simulink model "simulacionPOLGEN"  (R2017b)
settings: Solver=VariableStepDiscrete  StartTime=0.0  StopTime=20  MaxStep=0.1  RelTol=1e-3
undefined symbols (not defined in the file): sigbuilder_block
settings Model: Creator=Ian  LastModifiedBy=Ian

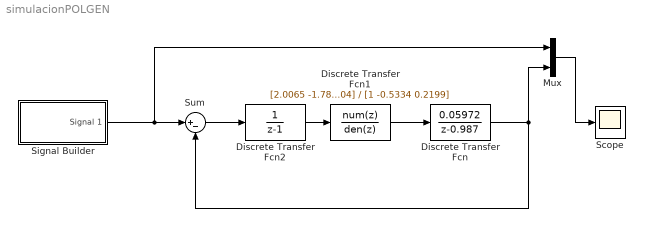
== system simulacionPOLGEN ==
  Discrete Transfer Fcn : DiscreteTransferFcn  Numerator=[0.05972]  Denominator=[1 -0.987]  SampleTime=0.1
  Discrete Transfer Fcn1 : DiscreteTransferFcn  Numerator=[2.0065 -1.7804]  Denominator=[1 -0.5334 0.2199]  SampleTime=0.1
  Discrete Transfer Fcn2 : DiscreteTransferFcn  Denominator=[1 -1]  SampleTime=0.1
  Mux : Mux  Inputs=2
  Scope : Scope
  Signal Builder : Subsystem  Tag=STV Subsys  LoadFcn=sigbuilder_block('load');  StartFcn=sigbuilder_block('start');  StopFcn=sigbuilder_block('stop');  ClipboardFcn=sigbuilder_block('clipboard');  mask(Sigbuilder block){tuvar=[0:10]}
      mask help: Simulink:masks:SigbuilderBlock_MD
      mask init:
      | if ~strcmp(get_param(bdroot(gcbh),'SimulationStatus'),'stopped') tuvar = sigbuilder_block('maskInit'); end
      settings: CopyFcn=sigbuilder_block('copy');  DeleteFcn=sigbuilder_block('delete');  ModelCloseFcn=sigbuilder_block('modelClose');  PreSaveFcn=sigbuilder_block('preSave');  PauseFcn=sigbuilder_block('pause');  ContinueFcn=sigbuilder_block('continue');  NameChangeFcn=sigbuilder_block('namechange');  OpenFcn=sigbuilder_block('open',[437.25 153 550.5 359.25 ]);  CloseFcn=sigbuilder_block('close');
      mask Display: plot(0, 0, 100, 100,[2, 2, 32, 32, 2], [68, 8, 8, 68, 68],[32, 2], [38, 38], [32, 19, 2],[53, 60, 44], [32, 17, 17, 2],[16, 16, 31, 31]);txt = getActiveGroup(gcbh);text(2, 100, txt,'verticalAlignment', 'top');
  Sum : Sum  Inputs=|+-
  wires:
  Discrete Transfer Fcn1/1 -> Discrete Transfer Fcn/1
  Discrete Transfer Fcn/1 -> Mux/2, Sum/2
  Signal Builder/1(Signal 1) -> Mux/1, Sum/1
  Mux/1 -> Scope/1
  Discrete Transfer Fcn2/1 -> Discrete Transfer Fcn1/1
  Sum/1 -> Discrete Transfer Fcn2/1

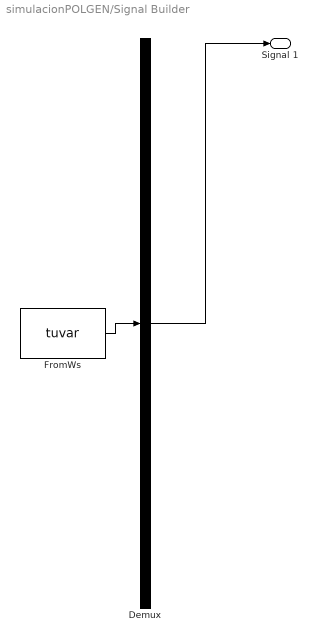
== system simulacionPOLGEN/Signal Builder ==
  Demux : Demux  Tag=STV Demux  Outputs=1
  FromWs : FromWorkspace  Tag=STV FromWs  VariableName=tuvar  SampleTime=0
      SigBuilderData=|
      | common.afterFinalStr = 'Extrapolate'
      | common.sampleTime = 0
      | dataSet.timeRange = [0 10]
      | dataSet.name = 'Group 1'
      | sbobj.Groups.Name = 'Group 1'
      | sbobj.Groups.Signals.Name = 'Signal 1'
      | sbobj.Groups.Signals.XData = [0 0.98 0.98 9.02 9.02 10]
      | sbobj.Groups.Signals.YData = [0 0 20 20 10 10]
  Signal 1 : Outport  Tag=STV Outport
  wires:
  Demux/1 -> Signal 1/1
  FromWs/1 -> Demux/1
